simulink model "encoder"  (R2022a)
settings: Solver=VariableStepAuto  StartTime=0.0  StopTime=10.0  RelTol=1e-3
settings Model: Creator=Matlab  LastModifiedBy=Matlab

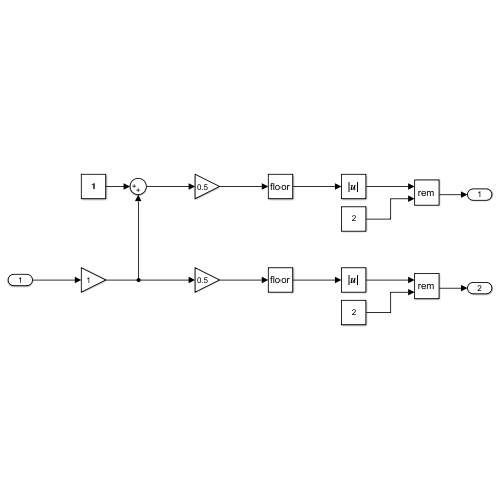
[thumbnail: Simulink's stored preview of the top-level diagram]
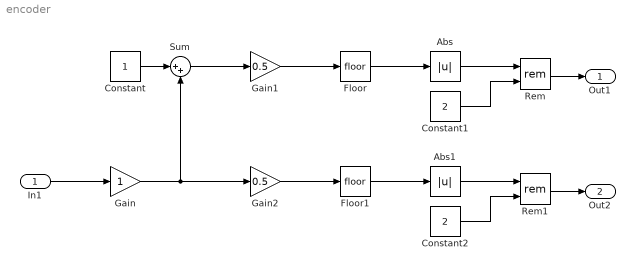
== system encoder ==
  In1 : Inport
  Abs : Abs  SaturateOnIntegerOverflow=off
  Abs1 : Abs  SaturateOnIntegerOverflow=off
  Constant : Constant
  Constant1 : Constant  Value=2
  Constant2 : Constant  Value=2
  Floor : Rounding
  Floor1 : Rounding
  Gain : Gain
  Gain1 : Gain  Gain=0.5
  Gain2 : Gain  Gain=0.5
  Rem : Math  Operator=rem
  Rem1 : Math  Operator=rem
  Sum : Sum  Inputs=|++
  Out1 : Outport
  Out2 : Outport  Port=2
  wires:
  Constant/1 -> Sum/1
  Gain/1 -> Sum/2, Gain2/1
  In1/1 -> Gain/1
  Sum/1 -> Gain1/1
  Gain1/1 -> Floor/1
  Gain2/1 -> Floor1/1
  Floor/1 -> Abs/1
  Floor1/1 -> Abs1/1
  Abs/1 -> Rem/1
  Constant1/1 -> Rem/2
  Rem/1 -> Out1/1
  Abs1/1 -> Rem1/1
  Constant2/1 -> Rem1/2
  Rem1/1 -> Out2/1
